simulink model "CruiseControl"  (R2020b)
settings: Solver=VariableStepAuto  StartTime=0.0  StopTime=10.0  RelTol=1e-3
undefined symbols (not defined in the file): b, m
settings Model: DataDictionary=CruiseControl.sldd  Creator=priyaD  LastModifiedBy=priyaD

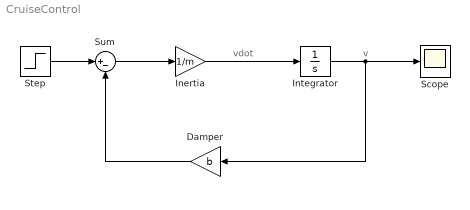
== system CruiseControl ==
  note: vdot
  note: v
  Damper : Gain  Gain=b
  Inertia : Gain  Gain=1/m
  Integrator : Integrator
  Scope : Scope
  Step : Step  SampleTime=0
  Sum : Sum  Inputs=|+-
  wires:
  Integrator/1 -> Scope/1, Damper/1
  Inertia/1 -> Integrator/1
  Sum/1 -> Inertia/1
  Damper/1 -> Sum/2
  Step/1 -> Sum/1
